simulink model "LinearSys2_org"  (Simulink 10.0)
settings: Solver=ode45  StartTime=0.0  StopTime=10  RelTol=1e-6  EnableMultiTasking=on
undefined symbols (not defined in the file): Ac, As, Bs, Cs, DiscIntNeverNeededParam, Ds, Filter_Coef, Gc, K_d, K_i, K_p, Kdf, Kdth, Kdy, Kith, Kiy, Kpth, Kpy, Mc, nullProj, omega_0, pinvBc, x0, xdes
libraries: dspstat3 x4, simulink x2
settings Model: Creator=nitisht  LastModifiedBy=annonymous  ExtModeTrigDuration=10000
settings DataIOCC: LimitDataPoints=on
settings OptimizationCC: ExpressionDepthLimit=2147483647
settings DebuggingCC: SolverPrmCheckMsg=warning  StateNameClashWarn=warning
settings HardwareCC: ProdIntDivRoundTo=Zero  ProdEndianess=LittleEndian  ProdHWDeviceType=Generic->32-bit x86 compatible  TargetBitPerLong=64  TargetBitPerPointer=64  TargetBitPerSizeT=64  TargetBitPerPtrDiffT=64  TargetLongLongMode=on  TargetIntDivRoundTo=Zero  TargetEndianess=LittleEndian  TargetWordSize=64  TargetHWDeviceType=MATLAB Host  ProdEqTarget=off
settings RTWCC: Description=Rapid Simulation Target  SystemTargetFile=rsim.tlc  TemplateMakefile=rsim_default_tmf  RTWCompilerOptimization=on
settings CodeAppCC: MaxIdLength=95
settings RSimTargetCC: PreserveStateflowLocalDataDimensions=off
settings ConfigComp: CovExternalEMLEnable=off

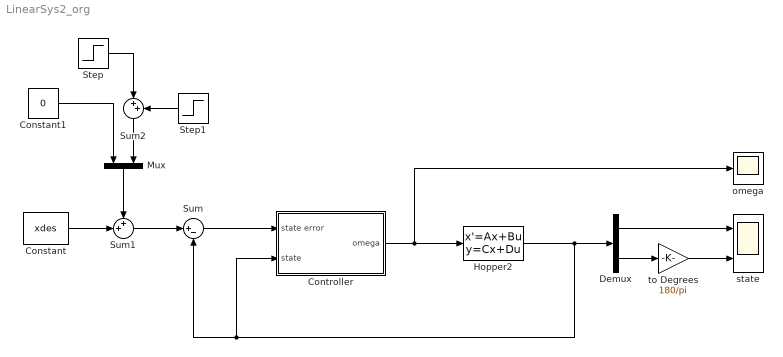
== system LinearSys2_org ==
  Constant : Constant  Value=xdes
  Constant1 : Constant  Value=0
  Controller : Subsystem
  Demux : Demux  Outputs=2
  Hopper2 : StateSpace  A=As  B=Bs  C=Cs  D=Ds  InitialCondition=x0
  Mux : Mux  Inputs=2
  Step : Step  Time=5  After=5*pi/180  SampleTime=0
  Step1 : Step  Time=10  After=-5*pi/180  SampleTime=0
  Sum : Sum  Inputs=|+-
  Sum1 : Sum  Inputs=++|
  Sum2 : Sum  Inputs=|++
  omega : Scope
  state : Scope  NumInputPorts=2
  to Degrees : Gain  Gain=180/pi
  wires:
  Hopper2/1 -> Demux/1, Controller/2(state), Sum/2
  Sum/1 -> Controller/1(state error)
  Demux/1 -> state/1
  Demux/2 -> to Degrees/1
  to Degrees/1 -> state/2
  Sum1/1 -> Sum/1
  Constant/1 -> Sum1/2
  Mux/1 -> Sum1/1
  Constant1/1 -> Mux/1
  Sum2/1 -> Mux/2
  Step/1 -> Sum2/1
  Step1/1 -> Sum2/2
  Controller/1(omega) -> Hopper2/1, omega/1

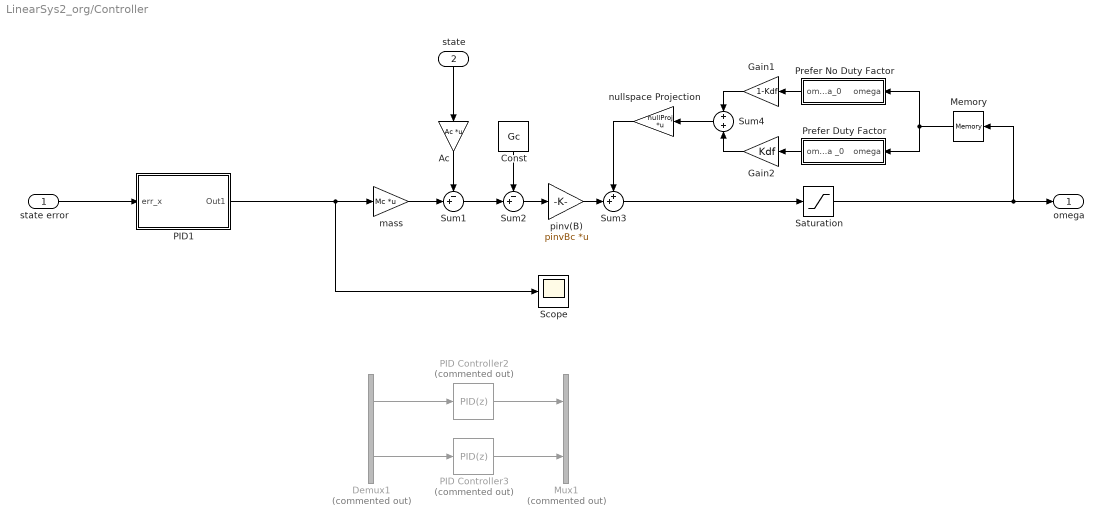
== system LinearSys2_org/Controller ==
  state error : Inport
  state : Inport  Port=2
  Ac : Gain  Gain=Ac  Multiplication=Matrix(K*u)
  Const : Constant  Value=Gc
  Demux1 : Demux  Commented=on  Outputs=2
  Gain1 : Gain  Gain=1-Kdf
  Gain2 : Gain  Gain=Kdf
  Memory : Memory  InitialCondition=omega_0  InheritSampleTime=on
  Mux1 : Mux  Commented=on  Inputs=2
  PID Controller2 : simulink/Continuous/PID Controller  Commented=on  Controller=PID  TimeDomain=Discrete-time  SampleTime=.01  IntegratorMethod=Forward Euler  FilterMethod=Forward Euler  Form=Parallel  P=Kpy  I=Kiy  D=Kdy  N=1000  InitialConditionSource=internal  InitialConditionForIntegrator=0  InitialConditionForFilter=0  ExternalReset=none  LimitOutput=off  UpperSaturationLimit=inf  LowerSaturationLimit=-inf  LinearizeAsGain=on  AntiWindupMode=none  Kb=1  TrackingMode=off  Kt=1  PParamMin=[]  PParamMax=[]  IParamMin=[]  IParamMax=[]  DParamMin=[]  DParamMax=[]  NParamMin=[]  NParamMax=[]  KbParamMin=[]  KbParamMax=[]  KtParamMin=[]  KtParamMax=[]  POutMin=[]  POutMax=[]  IOutMin=[]  IOutMax=[]  DOutMin=[]  DOutMax=[]  NOutMin=[]  NOutMax=[]  KbOutMin=[]  KbOutMax=[]  KtOutMin=[]  KtOutMax=[]  IntegratorOutMin=[]  IntegratorOutMax=[]  FilterOutMin=[]  FilterOutMax=[]  SumOutMin=[]  SumOutMax=[]  SumI1OutMin=[]  SumI1OutMax=[]  SumI2OutMin=[]  SumI2OutMax=[]  SumI3OutMin=[]  SumI3OutMax=[]  SumDOutMin=[]  SumDOutMax=[]  SaturationOutMin=[]  SaturationOutMax=[]  IntegratorContinuousStateAttributes=''  IntegratorStateMustResolveToSignalObject=off  IntegratorRTWStateStorageClass=Auto  FilterContinuousStateAttributes=''  FilterStateMustResolveToSignalObject=off  FilterRTWStateStorageClass=Auto
  PID Controller3 : simulink/Continuous/PID Controller  Commented=on  Controller=PID  TimeDomain=Discrete-time  SampleTime=.01  IntegratorMethod=Forward Euler  FilterMethod=Forward Euler  Form=Parallel  P=Kpth  I=Kith  D=Kdth  N=1000  InitialConditionSource=internal  InitialConditionForIntegrator=0  InitialConditionForFilter=0  ExternalReset=none  LimitOutput=off  UpperSaturationLimit=inf  LowerSaturationLimit=-inf  LinearizeAsGain=on  AntiWindupMode=none  Kb=1  TrackingMode=off  Kt=1  PParamMin=[]  PParamMax=[]  IParamMin=[]  IParamMax=[]  DParamMin=[]  DParamMax=[]  NParamMin=[]  NParamMax=[]  KbParamMin=[]  KbParamMax=[]  KtParamMin=[]  KtParamMax=[]  POutMin=[]  POutMax=[]  IOutMin=[]  IOutMax=[]  DOutMin=[]  DOutMax=[]  NOutMin=[]  NOutMax=[]  KbOutMin=[]  KbOutMax=[]  KtOutMin=[]  KtOutMax=[]  IntegratorOutMin=[]  IntegratorOutMax=[]  FilterOutMin=[]  FilterOutMax=[]  SumOutMin=[]  SumOutMax=[]  SumI1OutMin=[]  SumI1OutMax=[]  SumI2OutMin=[]  SumI2OutMax=[]  SumI3OutMin=[]  SumI3OutMax=[]  SumDOutMin=[]  SumDOutMax=[]  SaturationOutMin=[]  SaturationOutMax=[]  IntegratorContinuousStateAttributes=''  IntegratorStateMustResolveToSignalObject=off  IntegratorRTWStateStorageClass=Auto  FilterContinuousStateAttributes=''  FilterStateMustResolveToSignalObject=off  FilterRTWStateStorageClass=Auto
  PID1 : Subsystem  mask{P=K_p, I=K_i, D=K_d, N=Filter_Coef}
      mask prompts: P "Proportional Gain"; I "Integral Gain"; D "Derivative Gain"; N "Filter Coefficient"
  Prefer Duty Factor : Subsystem
  Prefer No Duty Factor : Subsystem
  Saturation : Saturate  UpperLimit=100  LowerLimit=10
  Scope : Scope
  Sum1 : Sum  Inputs=-+|
  Sum2 : Sum  Inputs=-+|
  Sum3 : Sum  Inputs=++|
  Sum4 : Sum  Inputs=+|+
  mass : Gain  Gain=Mc  Multiplication=Matrix(K*u)
  nullspace Projection : Gain  Gain=nullProj  Multiplication=Matrix(K*u)
  pinv(B) : Gain  Gain=pinvBc  Multiplication=Matrix(K*u)
  omega : Outport
  wires:
  Gain2/1 -> Sum4/2
  state/1 -> Ac/1
  Sum2/1 -> pinv(B)/1
  mass/1 -> Sum1/2
  Memory/1 -> Prefer No Duty Factor/1(omega), Prefer Duty Factor/1(omega)
  Gain1/1 -> Sum4/1
  Sum3/1 -> Saturation/1
  Sum4/1 -> nullspace Projection/1
  Saturation/1 -> Memory/1, omega/1
  Ac/1 -> Sum1/1
  pinv(B)/1 -> Sum3/2
  Sum1/1 -> Sum2/2
  Const/1 -> Sum2/1
  Prefer No Duty Factor/1(omega_0) -> Gain1/1
  Prefer Duty Factor/1(omega _0) -> Gain2/1
  nullspace Projection/1 -> Sum3/1
  PID Controller2/1 -> Mux1/1
  PID Controller3/1 -> Mux1/2
  Demux1/1 -> PID Controller2/1
  Demux1/2 -> PID Controller3/1
  PID1/1(Out1) -> Scope/1, mass/1
  state error/1 -> PID1/1(err_x)

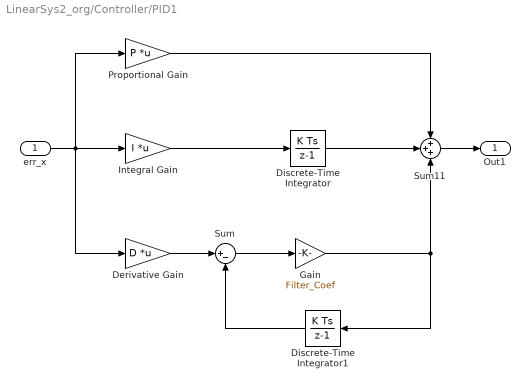
== system LinearSys2_org/Controller/PID1 ==
  err_x : Inport
  Derivative Gain : Gain  Gain=D  Multiplication=Matrix(K*u)
  Discrete-Time Integrator : DiscreteIntegrator  SampleTime=.01  ICPrevOutput=DiscIntNeverNeededParam  ICPrevScaledInput=DiscIntNeverNeededParam
  Discrete-Time Integrator1 : DiscreteIntegrator  SampleTime=.01  ICPrevOutput=DiscIntNeverNeededParam  ICPrevScaledInput=DiscIntNeverNeededParam
  Gain : Gain  Gain=Filter_Coef
  Integral Gain : Gain  DisableCoverage=on  Gain=I  Multiplication=Matrix(K*u)
  Proportional Gain : Gain  Gain=P  Multiplication=Matrix(K*u)
  Sum : Sum  Inputs=|+-
  Sum11 : Sum  Inputs=+++
  Out1 : Outport
  wires:
  Integral Gain/1 -> Discrete-Time Integrator/1
  Discrete-Time Integrator1/1 -> Sum/2
  Sum/1 -> Gain/1
  Derivative Gain/1 -> Sum/1
  err_x/1 -> Proportional Gain/1, Integral Gain/1, Derivative Gain/1
  Gain/1 -> Sum11/3, Discrete-Time Integrator1/1
  Discrete-Time Integrator/1 -> Sum11/2
  Sum11/1 -> Out1/1
  Proportional Gain/1 -> Sum11/1

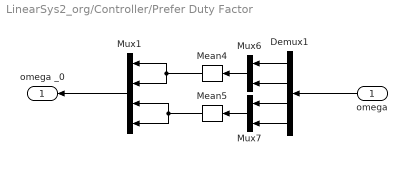
== system LinearSys2_org/Controller/Prefer Duty Factor ==
  omega : Inport
  Demux1 : Demux
  Mean4 : dspstat3/Mean  run=off  reset_popup=None  InputProcessing=Columns as channels (frame based)  directionMode=Each column  dimension=1  treatSBRowAsCol=on  roiEnable=off  roiType=Rectangles  roiPortion=Entire ROI  roiOutput=Individual statistics for each ROI  roiFlag=off  outputDataTypeStr=Inherit: Same as accumulator  outputLastDataTypeStr=Inherit: Same as accumulator  outputMin=[]  outputMax=[]  roundingMode=Floor  overflowMode=off
  Mean5 : dspstat3/Mean  run=off  reset_popup=None  InputProcessing=Columns as channels (frame based)  directionMode=Each column  dimension=1  treatSBRowAsCol=on  roiEnable=off  roiType=Rectangles  roiPortion=Entire ROI  roiOutput=Individual statistics for each ROI  roiFlag=off  outputDataTypeStr=Inherit: Same as accumulator  outputLastDataTypeStr=Inherit: Same as accumulator  outputMin=[]  outputMax=[]  roundingMode=Floor  overflowMode=off
  Mux1 : Mux
  Mux6 : Mux  Inputs=2
  Mux7 : Mux  Inputs=2
  omega _0 : Outport
  wires:
  Mean5/1 -> Mux1/3, Mux1/4
  Demux1/4 -> Mux7/2
  Demux1/3 -> Mux7/1
  Demux1/2 -> Mux6/2
  Mux6/1 -> Mean4/1
  Mux7/1 -> Mean5/1
  omega/1 -> Demux1/1
  Demux1/1 -> Mux6/1
  Mux1/1 -> omega _0/1
  Mean4/1 -> Mux1/1, Mux1/2

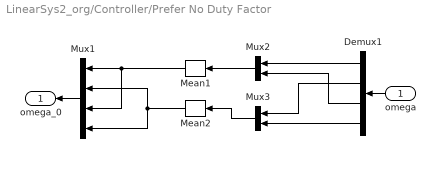
== system LinearSys2_org/Controller/Prefer No Duty Factor ==
  omega : Inport
  Demux1 : Demux
  Mean1 : dspstat3/Mean  run=off  reset_popup=None  InputProcessing=Columns as channels (frame based)  directionMode=Each column  dimension=1  treatSBRowAsCol=on  roiEnable=off  roiType=Rectangles  roiPortion=Entire ROI  roiOutput=Individual statistics for each ROI  roiFlag=off  outputDataTypeStr=Inherit: Same as accumulator  outputLastDataTypeStr=Inherit: Same as accumulator  outputMin=[]  outputMax=[]  roundingMode=Floor  overflowMode=off
  Mean2 : dspstat3/Mean  run=off  reset_popup=None  InputProcessing=Columns as channels (frame based)  directionMode=Each column  dimension=1  treatSBRowAsCol=on  roiEnable=off  roiType=Rectangles  roiPortion=Entire ROI  roiOutput=Individual statistics for each ROI  roiFlag=off  outputDataTypeStr=Inherit: Same as accumulator  outputLastDataTypeStr=Inherit: Same as accumulator  outputMin=[]  outputMax=[]  roundingMode=Floor  overflowMode=off
  Mux1 : Mux
  Mux2 : Mux  Inputs=2
  Mux3 : Mux  Inputs=2
  omega_0 : Outport
  wires:
  Demux1/4 -> Mux3/2
  Demux1/3 -> Mux2/2
  Mean2/1 -> Mux1/4, Mux1/2
  omega/1 -> Demux1/1
  Mean1/1 -> Mux1/1, Mux1/3
  Mux1/1 -> omega_0/1
  Demux1/2 -> Mux3/1
  Mux3/1 -> Mean2/1
  Mux2/1 -> Mean1/1
  Demux1/1 -> Mux2/1
